simulink model "ssc_battery_management_R2019b"  (R2019b)
settings: Solver=daessc  StartTime=0.0  StopTime=2000  FixedStep=0.1  MinStep=1e-6  RelTol=1e-5  EnableMultiTasking=on
PreLoadFcn:
  | ModelPath = fileparts(get_param(bdroot,'FileName'));
  | addpath(ModelPath);
  | 
  | ssc_battery_management_R2012b_ini
values from neighbouring files (symbols this model uses):
  AltData100AMaxCurrent =     [AlternatorTableData.mat]
  AltData100AVoltage =     [AlternatorTableData.mat]
  AltData80AMaxCurrent =     [AlternatorTableData.mat]
  AltData80AVoltage =     [AlternatorTableData.mat]
  Kt = [0.80,1.10,1.20,1.12;]    [ssc_lead_acid_battery_50Ah_ini.m]    (also in ssc_lead_acid_battery_80Ah_ini.m)
  Kt_Temps = [25 40 60 75]    [ssc_lead_acid_battery_50Ah_ini.m]    (also in ssc_lead_acid_battery_80Ah_ini.m)
  theta_f = -40    [ssc_lead_acid_battery_50Ah_ini.m]    (also in ssc_lead_acid_battery_80Ah_ini.m)
  theta_init = 25    [ssc_lead_acid_battery_50Ah_ini.m]    (also in ssc_lead_acid_battery_80Ah_ini.m)
undefined symbols (not defined in the file or in its folder): beta, center, DiscIntNeverNeededParam, exponent, polyTerms, sigbuilder_block, WendlandNumTerms, width
libraries: fl_lib x130, LeadAcidBattery_lib x36, nesl_utility x28, simulink x6
(part 4 of 4)

== system ssc_battery_management_R2019b/Alternator Variants/Alternator_80A_MBC/Alternator/80A_Max_Current/Constraint Block/Constraints/Constraint ==
  Xin : Inport
  Constraint - conrange : Subsystem  mask(Range Constraint){}
      mask help: This block impements range constraints for MBC models
      mask init:
      | ud = get_param( gcb, 'UserData' );M = ud.M;HW = ud.HW;LB = ud.LB;UB = ud.UB;Scale = ud.Scale;
  switch : Switch  SaturateOnIntegerOverflow=on  InputSameDT=on
  Distance : Outport
  Interior Point : Outport  Port=2
  wires:
  Constraint - conrange/2(Interior Point) -> switch/1
  Constraint - conrange/1(Distance) -> switch/2, Distance/1
  Xin/1 -> Constraint - conrange/1(Xin), switch/3
  switch/1 -> Interior Point/1

== system ssc_battery_management_R2019b/Alternator Variants/Alternator_80A_MBC/Alternator/80A_Max_Current/xregrbf/rbflogisticrbfEval/Logistic ==
  R/S : Inport
  Constant5 : Constant
  Math Function1 : Math  Operator=reciprocal  SaturateOnIntegerOverflow=on
  Math Function2 : Math  SaturateOnIntegerOverflow=on
  Sum1 : Sum  Inputs=|++  SaturateOnIntegerOverflow=on  InputSameDT=on  OutDataTypeStr=Inherit: Same as first input
  P : Outport
  wires:
  Math Function1/1 -> P/1
  Sum1/1 -> Math Function1/1
  Constant5/1 -> Sum1/2
  Math Function2/1 -> Sum1/1
  R/S/1 -> Math Function2/1

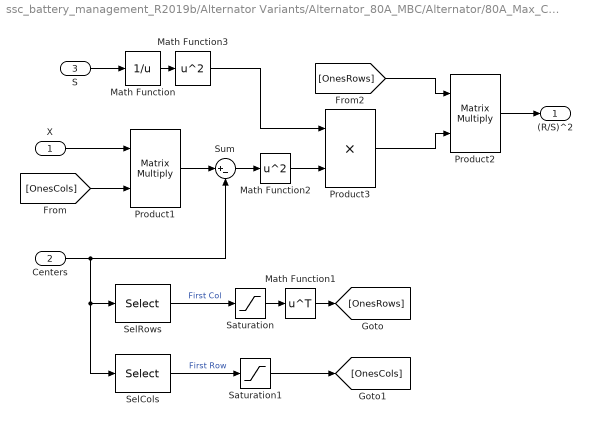
== system ssc_battery_management_R2019b/Alternator Variants/Alternator_80A_MBC/Alternator/80A_Max_Current/xregrbf/rbflogisticrbfEval/R ==
  X : Inport
  "Centers " : Inport  Port=2
  S : Inport  Port=3
  Math Function : Math  Operator=reciprocal  SaturateOnIntegerOverflow=on
  Math Function1 : Math  Operator=transpose  SaturateOnIntegerOverflow=on
  Math Function2 : Math  Operator=square  SaturateOnIntegerOverflow=on
  Math Function3 : Math  Operator=square  SaturateOnIntegerOverflow=on
  Product1 : Product  Multiplication=Matrix(*)  SaturateOnIntegerOverflow=on  InputSameDT=on  OutDataTypeStr=Inherit: Same as first input
  Product2 : Product  Multiplication=Matrix(*)  SaturateOnIntegerOverflow=on  InputSameDT=on  OutDataTypeStr=Inherit: Same as first input
  Product3 : Product  SaturateOnIntegerOverflow=on  InputSameDT=on  OutDataTypeStr=Inherit: Same as first input
  Saturation : Saturate  UpperLimit=1  LowerLimit=1
  Saturation1 : Saturate  UpperLimit=1  LowerLimit=1
  SelCols : Selector  NumberOfDimensions=2  InputPortWidth=3  IndexOptions=Index vector (dialog),Select all  Indices=1,-1  OutputSizes=1
  SelRows : Selector  NumberOfDimensions=2  InputPortWidth=3  IndexOptions=Select all,Index vector (dialog)  Indices=-1,1  OutputSizes=1
  Sum : Sum  Inputs=|+-  SaturateOnIntegerOverflow=on  InputSameDT=on  OutDataTypeStr=Inherit: Same as first input
  (R/S)^2 : Outport
  wires:
  Math Function2/1 -> Product3/2
  Sum/1 -> Math Function2/1
  Product1/1 -> Sum/1
  X/1 -> Product1/1
  [OnesCols] -> Product1/2
  Math Function1/1 -> [OnesRows]
  SelRows/1 -> Saturation/1  "First Col"
  "Centers "/1 -> Sum/2, SelRows/1, SelCols/1
  S/1 -> Math Function/1
  Math Function/1 -> Math Function3/1
  Saturation/1 -> Math Function1/1
  SelCols/1 -> Saturation1/1  "First Row"
  Saturation1/1 -> [OnesCols]
  Math Function3/1 -> Product3/1
  Product3/1 -> Product2/2
  Product2/1 -> (R/S)^2/1
  [OnesRows] -> Product2/1

== system ssc_battery_management_R2019b/Alternator Variants/Alternator_80A_MBC/Alternator/80A_Voltage/Constraint Block/Constraints/Constraint ==
  Xin : Inport
  Constraint - conrange : Subsystem  mask(Range Constraint){}
      mask help: This block impements range constraints for MBC models
      mask init:
      | ud = get_param( gcb, 'UserData' );M = ud.M;HW = ud.HW;LB = ud.LB;UB = ud.UB;Scale = ud.Scale;
  switch : Switch  SaturateOnIntegerOverflow=on  InputSameDT=on
  Distance : Outport
  Interior Point : Outport  Port=2
  wires:
  Constraint - conrange/2(Interior Point) -> switch/1
  Constraint - conrange/1(Distance) -> switch/2, Distance/1
  Xin/1 -> Constraint - conrange/1(Xin), switch/3
  switch/1 -> Interior Point/1

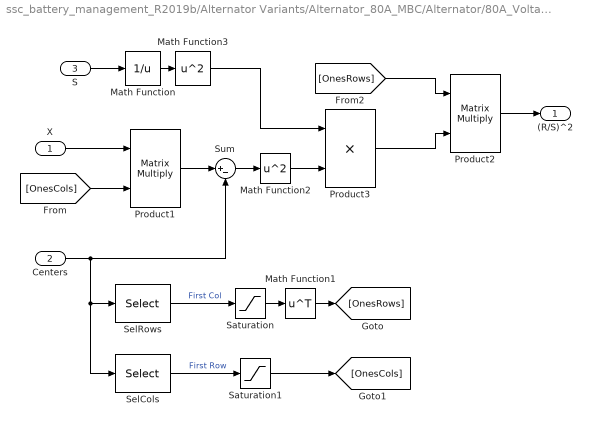
== system ssc_battery_management_R2019b/Alternator Variants/Alternator_80A_MBC/Alternator/80A_Voltage/xregrbf/rbfwendlandEval/R ==
  X : Inport
  "Centers " : Inport  Port=2
  S : Inport  Port=3
  Math Function : Math  Operator=reciprocal  SaturateOnIntegerOverflow=on
  Math Function1 : Math  Operator=transpose  SaturateOnIntegerOverflow=on
  Math Function2 : Math  Operator=square  SaturateOnIntegerOverflow=on
  Math Function3 : Math  Operator=square  SaturateOnIntegerOverflow=on
  Product1 : Product  Multiplication=Matrix(*)  SaturateOnIntegerOverflow=on  InputSameDT=on  OutDataTypeStr=Inherit: Same as first input
  Product2 : Product  Multiplication=Matrix(*)  SaturateOnIntegerOverflow=on  InputSameDT=on  OutDataTypeStr=Inherit: Same as first input
  Product3 : Product  SaturateOnIntegerOverflow=on  InputSameDT=on  OutDataTypeStr=Inherit: Same as first input
  Saturation : Saturate  UpperLimit=1  LowerLimit=1
  Saturation1 : Saturate  UpperLimit=1  LowerLimit=1
  SelCols : Selector  NumberOfDimensions=2  InputPortWidth=3  IndexOptions=Index vector (dialog),Select all  Indices=1,-1  OutputSizes=1
  SelRows : Selector  NumberOfDimensions=2  InputPortWidth=3  IndexOptions=Select all,Index vector (dialog)  Indices=-1,1  OutputSizes=1
  Sum : Sum  Inputs=|+-  SaturateOnIntegerOverflow=on  InputSameDT=on  OutDataTypeStr=Inherit: Same as first input
  (R/S)^2 : Outport
  wires:
  Math Function2/1 -> Product3/2
  Sum/1 -> Math Function2/1
  Product1/1 -> Sum/1
  X/1 -> Product1/1
  [OnesCols] -> Product1/2
  Math Function1/1 -> [OnesRows]
  SelRows/1 -> Saturation/1  "First Col"
  "Centers "/1 -> Sum/2, SelRows/1, SelCols/1
  S/1 -> Math Function/1
  Math Function/1 -> Math Function3/1
  Saturation/1 -> Math Function1/1
  SelCols/1 -> Saturation1/1  "First Row"
  Saturation1/1 -> [OnesCols]
  Math Function3/1 -> Product3/1
  Product3/1 -> Product2/2
  Product2/1 -> (R/S)^2/1
  [OnesRows] -> Product2/1

== system ssc_battery_management_R2019b/Alternator Variants/Alternator_80A_MBC/Alternator/80A_Voltage/xregrbf/rbfwendlandEval/Wendland ==
  R/S : Inport
  PolyTerms : Inport  Port=2
  Exponent : Inport  Port=3
  Constant : Constant
  Constant1 : Constant  Value=0
  Math Function1 : Math  Operator=pow  SaturateOnIntegerOverflow=on
  Product : Product  SaturateOnIntegerOverflow=on  InputSameDT=on  OutDataTypeStr=Inherit: Same as first input
  S-Function : S-Function  FunctionName=WendlandEvalSFnV1  Parameters=NumTerms  SFunctionDeploymentMode=off  EnableBusSupport=off
  Sum : Sum  Inputs=-+|  SaturateOnIntegerOverflow=on  InputSameDT=on  OutDataTypeStr=Inherit: Same as first input
  Switch : Switch  InputSameDT=on
  P : Outport
  wires:
  Product/1 -> P/1
  R/S/1 -> S-Function/2, Sum/1  "R/S"
  PolyTerms/1 -> S-Function/1
  Constant/1 -> Sum/2
  Exponent/1 -> Math Function1/2
  Constant1/1 -> Switch/3
  S-Function/1 -> Product/1
  Sum/1 -> Math Function1/1, Switch/2
  Math Function1/1 -> Switch/1
  Switch/1 -> Product/2

== system ssc_battery_management_R2019b/Alternator Variants/Alternator_100A_MBC/Alternator/100A_Max_Current/Constraint Block/Constraints/Constraint/Constraint - conrange ==
  note: M = (UB+LB)/2
      | HW = (UB-LB)/2
  Xin : Inport
  Abs : Abs  SaturateOnIntegerOverflow=on
  Gain1 : Gain  Gain=Scale  SaturateOnIntegerOverflow=on  OutDataTypeStr=Inherit: Same as input  ParamDataTypeStr=Inherit: Same as input
  Half width : Constant  Value=HW
  Lower bounds : Constant  Value=LB
  Mid-point : Constant  Value=M
  Sum : Sum  Inputs=|+-  SaturateOnIntegerOverflow=on
  Sum1 : Sum  Inputs=|+-  SaturateOnIntegerOverflow=on
  Upper bounds : Constant  Value=UB
  max : MinMax  Function=max  Inputs=2  SaturateOnIntegerOverflow=on  InputSameDT=on
  max1 : MinMax  Function=max  SaturateOnIntegerOverflow=on  InputSameDT=on
  min : MinMax  Inputs=2  SaturateOnIntegerOverflow=on  InputSameDT=on
  Distance : Outport
  Interior Point : Outport  Port=2
  wires:
  Xin/1 -> max/2, Sum/1
  max1/1 -> Distance/1
  Sum1/1 -> Gain1/1
  Half width/1 -> Sum1/2
  Abs/1 -> Sum1/1
  Sum/1 -> Abs/1
  Mid-point/1 -> Sum/2
  min/1 -> Interior Point/1
  Upper bounds/1 -> min/2
  max/1 -> min/1
  Lower bounds/1 -> max/1
  Gain1/1 -> max1/1

== system ssc_battery_management_R2019b/Alternator Variants/Alternator_100A_MBC/Alternator/100A_Voltage/Constraint Block/Constraints/Constraint/Constraint - conrange ==
  note: M = (UB+LB)/2
      | HW = (UB-LB)/2
  Xin : Inport
  Abs : Abs  SaturateOnIntegerOverflow=on
  Gain1 : Gain  Gain=Scale  SaturateOnIntegerOverflow=on  OutDataTypeStr=Inherit: Same as input  ParamDataTypeStr=Inherit: Same as input
  Half width : Constant  Value=HW
  Lower bounds : Constant  Value=LB
  Mid-point : Constant  Value=M
  Sum : Sum  Inputs=|+-  SaturateOnIntegerOverflow=on
  Sum1 : Sum  Inputs=|+-  SaturateOnIntegerOverflow=on
  Upper bounds : Constant  Value=UB
  max : MinMax  Function=max  Inputs=2  SaturateOnIntegerOverflow=on  InputSameDT=on
  max1 : MinMax  Function=max  SaturateOnIntegerOverflow=on  InputSameDT=on
  min : MinMax  Inputs=2  SaturateOnIntegerOverflow=on  InputSameDT=on
  Distance : Outport
  Interior Point : Outport  Port=2
  wires:
  Xin/1 -> max/2, Sum/1
  max1/1 -> Distance/1
  Sum1/1 -> Gain1/1
  Half width/1 -> Sum1/2
  Abs/1 -> Sum1/1
  Sum/1 -> Abs/1
  Mid-point/1 -> Sum/2
  min/1 -> Interior Point/1
  Upper bounds/1 -> min/2
  max/1 -> min/1
  Lower bounds/1 -> max/1
  Gain1/1 -> max1/1

== system ssc_battery_management_R2019b/Alternator Variants/Alternator_80A_MBC/Alternator/80A_Max_Current/Constraint Block/Constraints/Constraint/Constraint - conrange ==
  note: M = (UB+LB)/2
      | HW = (UB-LB)/2
  Xin : Inport
  Abs : Abs  SaturateOnIntegerOverflow=on
  Gain1 : Gain  Gain=Scale  SaturateOnIntegerOverflow=on  OutDataTypeStr=Inherit: Same as input  ParamDataTypeStr=Inherit: Same as input
  Half width : Constant  Value=HW
  Lower bounds : Constant  Value=LB
  Mid-point : Constant  Value=M
  Sum : Sum  Inputs=|+-  SaturateOnIntegerOverflow=on
  Sum1 : Sum  Inputs=|+-  SaturateOnIntegerOverflow=on
  Upper bounds : Constant  Value=UB
  max : MinMax  Function=max  Inputs=2  SaturateOnIntegerOverflow=on  InputSameDT=on
  max1 : MinMax  Function=max  SaturateOnIntegerOverflow=on  InputSameDT=on
  min : MinMax  Inputs=2  SaturateOnIntegerOverflow=on  InputSameDT=on
  Distance : Outport
  Interior Point : Outport  Port=2
  wires:
  Xin/1 -> max/2, Sum/1
  max1/1 -> Distance/1
  Sum1/1 -> Gain1/1
  Half width/1 -> Sum1/2
  Abs/1 -> Sum1/1
  Sum/1 -> Abs/1
  Mid-point/1 -> Sum/2
  min/1 -> Interior Point/1
  Upper bounds/1 -> min/2
  max/1 -> min/1
  Lower bounds/1 -> max/1
  Gain1/1 -> max1/1

== system ssc_battery_management_R2019b/Alternator Variants/Alternator_80A_MBC/Alternator/80A_Voltage/Constraint Block/Constraints/Constraint/Constraint - conrange ==
  note: M = (UB+LB)/2
      | HW = (UB-LB)/2
  Xin : Inport
  Abs : Abs  SaturateOnIntegerOverflow=on
  Gain1 : Gain  Gain=Scale  SaturateOnIntegerOverflow=on  OutDataTypeStr=Inherit: Same as input  ParamDataTypeStr=Inherit: Same as input
  Half width : Constant  Value=HW
  Lower bounds : Constant  Value=LB
  Mid-point : Constant  Value=M
  Sum : Sum  Inputs=|+-  SaturateOnIntegerOverflow=on
  Sum1 : Sum  Inputs=|+-  SaturateOnIntegerOverflow=on
  Upper bounds : Constant  Value=UB
  max : MinMax  Function=max  Inputs=2  SaturateOnIntegerOverflow=on  InputSameDT=on
  max1 : MinMax  Function=max  SaturateOnIntegerOverflow=on  InputSameDT=on
  min : MinMax  Inputs=2  SaturateOnIntegerOverflow=on  InputSameDT=on
  Distance : Outport
  Interior Point : Outport  Port=2
  wires:
  Xin/1 -> max/2, Sum/1
  max1/1 -> Distance/1
  Sum1/1 -> Gain1/1
  Half width/1 -> Sum1/2
  Abs/1 -> Sum1/1
  Sum/1 -> Abs/1
  Mid-point/1 -> Sum/2
  min/1 -> Interior Point/1
  Upper bounds/1 -> min/2
  max/1 -> min/1
  Lower bounds/1 -> max/1
  Gain1/1 -> max1/1

== stateflow chart ssc_battery_management_R2019b/RPM Compensation/RPM Compensation- ALT Duty ==
  settings: updateMethod=DISCRETE  sampleTime=1
  state Increase
  state Normal
  state Decrease
  Increase -> (junction 16) [order 1] : [after(60,tick)]
  (junction 16) -> (junction 15) : {
      | step++;
      | }
  Increase -> Normal [order 2] : [before(60,tick) && Duty < DutyLimit[2]]
  Normal -> Increase [order 1] : [step<5 && Duty>DutyLimit[2]]
  (default) -> Normal
  (junction 15) -> Normal : {
      | RPM_comp = step * RPM_step;
      | }
  (junction 14) -> (junction 15) : {
      | step--;
      | }
  Decrease -> Normal [order 1] : [before(120,tick) && Duty > DutyLimit[1]]
  Normal -> Decrease [order 2] : [step>0 && Duty<DutyLimit[1]]
  Decrease -> (junction 14) [order 2] : [after(120,tick)]
  data: Duty input; DutyLimit input size=2; RPM_comp output double; RPM_step input; step output int8

== stateflow chart ssc_battery_management_R2019b/RPM Compensation/RPM Compensation- Batt Voltage ==
  settings: updateMethod=DISCRETE  sampleTime=1
  (default) -> (junction 58)
  (junction 58) -> (junction 57) [order 1] : [Integral >= 12]
  (junction 58) -> (junction 50) [order 2]
  (junction 57) -> (junction 55)
  (junction 55) -> (junction 56) [order 1] : [step1_flag == 1]
  (junction 55) -> (junction 54) [order 2] : {
      | RPM_comp += RPM_step;
      | step1_flag =1;
      | }
  (junction 56) -> (junction 53)
  (junction 53) -> (junction 54)
  (junction 54) -> (junction 43)
  (junction 43) -> (junction 44) [order 1] : [Integral >= 18]
  (junction 43) -> (junction 49) [order 2]
  (junction 44) -> (junction 52)
  (junction 50) -> (junction 45) [order 1] : [step1_flag == 0]
  (junction 50) -> (junction 40) [order 2]
  (junction 45) -> (junction 60)
  (junction 49) -> (junction 47) [order 1] : [step2_flag == 1]
  (junction 49) -> (junction 48) [order 2]
  (junction 47) -> (junction 38)
  (junction 40) -> (junction 46) [order 1] : [Integral < 2]
  (junction 52) -> (junction 35) [order 1] : [step2_flag == 1]
  (junction 38) -> (junction 37) [order 1] : [Integral < 17]
  (junction 40) -> (junction 42) [order 2]
  (junction 46) -> (junction 41) : {
      | RPM_comp += RPM_step;
      | step1_flag = 0;
      | }
  (junction 52) -> (junction 36) [order 2] : {
      | RPM_comp += RPM_step;
      | step2_flag = 1;
      | }
  (junction 35) -> (junction 59)
  (junction 38) -> (junction 51) [order 2]
  (junction 37) -> (junction 39) : {
      | RPM_comp -= RPM_step;
      | step2_flag = 0;
      | }
  (junction 41) -> (junction 42)
  (junction 60) -> (junction 41)
  (junction 48) -> (junction 60)
  (junction 51) -> (junction 48)
  (junction 39) -> (junction 51)
  (junction 36) -> (junction 39)
  (junction 59) -> (junction 36)
  data: RPM_comp output double; step1_flag output boolean; step2_flag output boolean; Integral input; RPM_step input
